simulink model "mrac_2vars"  (R2018a)
settings: Solver=VariableStepAuto  StartTime=0.0  StopTime=100  MaxStep=1e-2  RelTol=1e-3
InitFcn:
  | am = 2.0;
  | bm = 2.0;
  | a = 1.0;
  | b = 0.5;
settings Model: Creator=saad  LastModifiedBy=saad

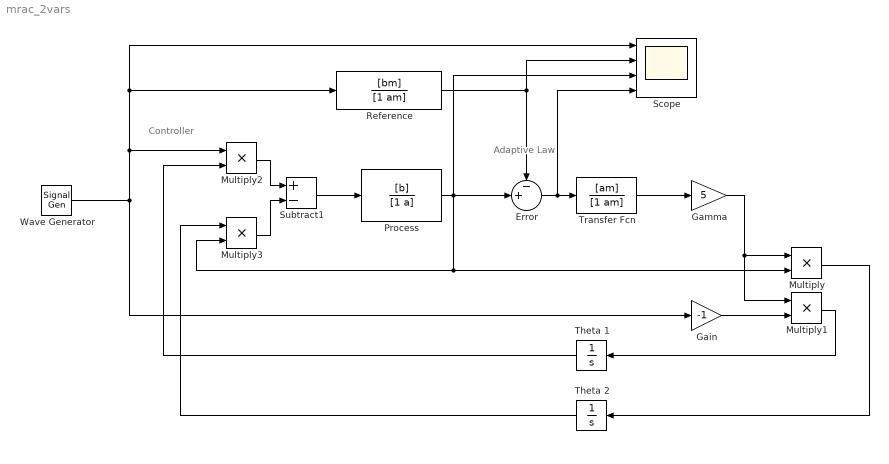
== system mrac_2vars ==
  note: Adaptive Law
  note: Controller
  Error : Sum  Inputs=-+|
  Gain : Gain  Gain=-1
  Gamma : Gain  Gain=5
  Multiply{,1..3} (4 alike) : Product
  Process : TransferFcn  Numerator=[b]  Denominator=[1 a]
  Reference : TransferFcn  Numerator=[bm]  Denominator=[1 am]
  "Scope " : Scope  NumInputPorts=4
  Subtract1 : Sum  Inputs=+-
  Theta 1 : Integrator
  Theta 2 : Integrator
  Transfer Fcn : TransferFcn  Numerator=[am]  Denominator=[1 am]
  Wave Generator : SignalGenerator  Amplitude=-1  Frequency=1/20
  wires:
  Wave Generator/1 -> Multiply2/1, "Scope "/1, Reference/1, Gain/1
  Process/1 -> Multiply3/2, Multiply/2, "Scope "/3, Error/2
  Reference/1 -> Error/1, "Scope "/2
  Error/1 -> "Scope "/4, Transfer Fcn/1
  Transfer Fcn/1 -> Gamma/1
  Gamma/1 -> Multiply/1, Multiply1/1
  Gain/1 -> Multiply1/2
  Multiply/1 -> Theta 2/1
  Multiply1/1 -> Theta 1/1
  Theta 1/1 -> Multiply2/2
  Theta 2/1 -> Multiply3/1
  Subtract1/1 -> Process/1
  Multiply2/1 -> Subtract1/1
  Multiply3/1 -> Subtract1/2
